simulink model "single_engine_neural_nn_predictive_260120"  (R2018b)
settings: Solver=VariableStepAuto  StartTime=0.0  StopTime=10.0  RelTol=1e-3
libraries: neural x1
settings Model: Creator=Paweł Tymiński  LastModifiedBy=Paweł Tymiński

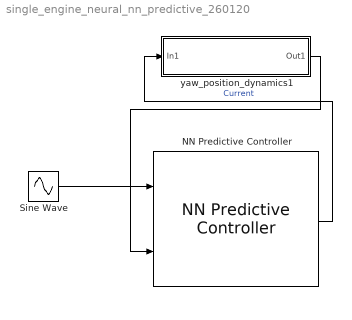
== system single_engine_neural_nn_predictive_260120 ==
  NN Predictive Controller : neural/Control Systems/NN Predictive Controller  epochs=1000  minp=-2.455060285275362908  maxp=2.495947464788551784  mint=-2.4550602852753495853  maxt=2.495947464788551784  Normalize=0  IW=[-0.00018471448141753606478 -0.018133954739487350566 0.0072916256365734861272 0.001695854239237938382;1.7928894707195155434 -1.969083405166670353 0.016675614316564738027 -0.036346866854253645496]  LW1_2=[-0.049855771222789169173 0.014670001734359346124 -0.00070480294703150370584 0.00020530021853124559247;-0.58787266159909246088 0.40744724440704482848 -0.25816189994354399317 0.069930134415343833676]  LW2_1=[-22.441360424601423773 0.018998459515510341539]  B1=[-0.0068409389362303445192;-0.07291783593751932635]  B2=-0.15207779069765531288  max_i_int=0  min_i_int=0  limit_output=0  max_output=0  min_output=0  Use_Previous_Weights=1  N2=4  Nu=5  Ts=0.001  rho=0.01  alpha=1  csrchfun=csrchbac  maxiter=1  S1=2  Ni=4  Nj=4  sim_file=0  trainfun=trainlm  Use_validation=1  Use_Testing=1  max_i=3  min_i=-3  sam_training=0
      settings: SourceProductName=Neural Network Toolbox  SourceProductBaseCode=NN
  Sine Wave : Sin  SampleTime=0
  yaw_position_dynamics1 : Subsystem
  wires:
  Sine Wave/1 -> NN Predictive Controller/1
  NN Predictive Controller/1 -> yaw_position_dynamics1/1(In1)  "Current"
  yaw_position_dynamics1/1(Out1) -> NN Predictive Controller/2

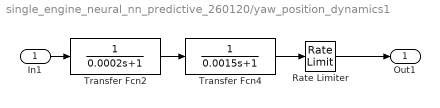
== system single_engine_neural_nn_predictive_260120/yaw_position_dynamics1 ==
  In1 : Inport
  Rate Limiter : RateLimiter  RisingSlewLimit=18.5  FallingSlewLimit=-18.5  SampleTimeMode=inherited
  Transfer Fcn2 : TransferFcn  Denominator=[0.0002 1]
  Transfer Fcn4 : TransferFcn  Denominator=[0.0015 1]
  Out1 : Outport
  wires:
  Transfer Fcn2/1 -> Transfer Fcn4/1
  In1/1 -> Transfer Fcn2/1
  Transfer Fcn4/1 -> Rate Limiter/1
  Rate Limiter/1 -> Out1/1
